simulink model "VA2_CV8_sim2017a"  (R2018a)
settings: Solver=ode45  StartTime=0.0  StopTime=3.5  RelTol=1e-3  EnableMultiTasking=on
values from neighbouring files (symbols this model uses):
  A = [ 0       1   0       0 ... (first row only)    [VA2_CV8_matlab_final.m]    (also in VA2_CV8_matlab_test.m)
  B = [0;    -0.0633;   0;   3.4960]    [VA2_CV8_matlab_final.m]    (also in VA2_CV8_matlab_test.m)
  C = eye(4)    [VA2_CV8_matlab_final.m]    (also in VA2_CV8_matlab_test.m)
  D = zeros(4,1)    [VA2_CV8_matlab_final.m]    (also in VA2_CV8_matlab_test.m)
  H = place(A', C', observer_poles)'    [VA2_CV8_matlab_final.m]
  Ki = -K(5)    [VA2_CV8_matlab_final.m]
  Kr = K(1:n)    [VA2_CV8_matlab_final.m]
  maxR = 7/weight    (= 1.29390018484)    [VA2_CV8_matlab_final.m]
libraries: sldrtlib x1
settings Model: Creator=pvel  LastModifiedBy=romanp
settings DataIOCC: LimitDataPoints=on  SaveFormat=Array
settings OptimizationCC: LifeSpan=inf
settings DebuggingCC: SFUnexpectedBacktrackingDiag=warning  SFNoUnconditionalDefaultTransitionDiag=warning  SFExecutionAtInitializationDiag=none
settings HardwareCC: ProdBitPerPointer=32  ProdBitPerSizeT=32  ProdBitPerPtrDiffT=32  ProdLargestAtomicFloat=None  ProdIntDivRoundTo=Undefined  ProdEndianess=Unspecified  ProdWordSize=32  ProdHWDeviceType=32-bit Generic
settings ModelReferenceCC: PropagateSignalLabelsOutOfModel=off
settings CodeAppCC: StateflowObjectComments=on
settings GRTTargetCC: TargetLangStandard=C89/C90 (ANSI)  GeneratePreprocessorConditionals=Disable all
settings ConfigComp: CovMetricSettings=dw  CovHtmlReporting=on  CovSaveCumulativeToWorkspaceVar=on  CovSaveSingleToWorkspaceVar=on  CovExternalEMLEnable=off

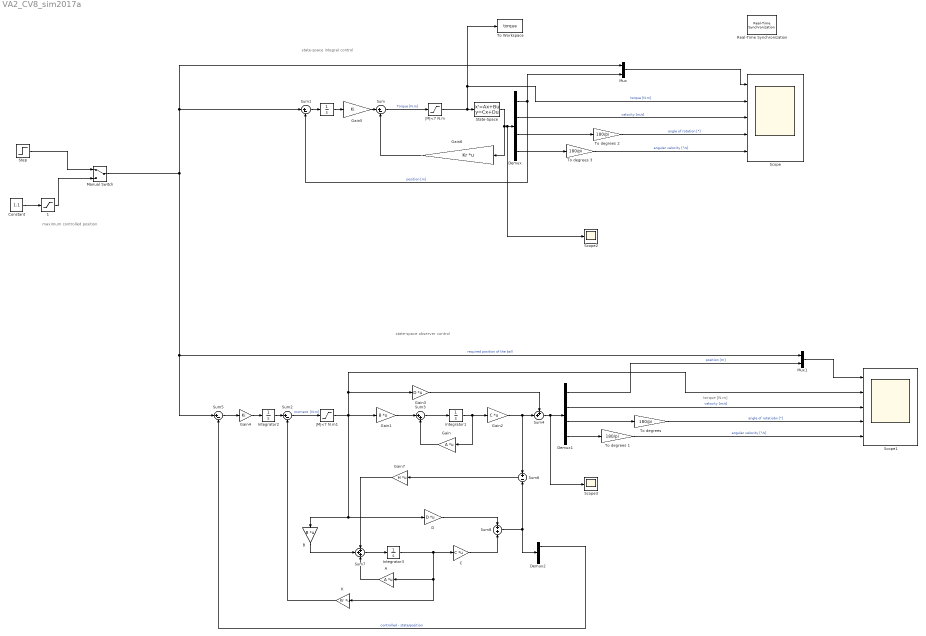
== system VA2_CV8_sim2017a ==
  note: torque [N.m]
  note: state-space integral control
  note: state-space observer control
  note: maximum controlled position
  " " : Integrator
  " 1" : Saturate  UpperLimit=maxR  LowerLimit=-maxR
  A : Gain  Gain=A  Multiplication=Matrix(K*u)
  B : Gain  Gain=B  Multiplication=Matrix(K*u)
  C : Gain  Gain=C  Multiplication=Matrix(K*u)
  Constant : Constant  Value=1.1
  "D " : Gain  Gain=D  Multiplication=Matrix(K*u)
  Demux : Demux
  Demux1 : Demux
  Demux2 : Demux
  Gain : Gain  Gain=A  Multiplication=Matrix(K*u)
  Gain1 : Gain  Gain=B  Multiplication=Matrix(K*u)
  Gain2 : Gain  Gain=C  Multiplication=Matrix(K*u)
  Gain3 : Gain  Gain=D  Multiplication=Matrix(K*u)
  Gain4 : Gain  Gain=Ki
  Gain5 : Gain  Gain=Ki
  Gain6 : Gain  Gain=Kr  Multiplication=Matrix(K*u) (u vector)
  Gain7 : Gain  Gain=H  Multiplication=Matrix(K*u)
  Integrator1 : Integrator
  Integrator2 : Integrator
  Integrator3 : Integrator
  K : Gain  Gain=Kr  Multiplication=Matrix(K*u)
  Manual Switch : ManualSwitch
  Mux : Mux  Inputs=2
  Mux1 : Mux  Inputs=2
  Real-Time Synchronization : sldrtlib/Real-Time Synchronization  SampleTime=0.1  MaxMissedTicks=10  ShowMissedTicks=off  YieldWhenWaiting=off
  Scope : Scope  NumInputPorts=5
  Scope1 : Scope  NumInputPorts=5
  Scope2 : Scope
  Scope3 : Scope
  State-Space : StateSpace  A=A  B=B  C=C  D=D  InitialCondition=0
  Step : Step  SampleTime=0
  Sum{,1..2,5} (4 alike) : Sum  Inputs=|+-
  Sum3 : Sum  Inputs=|++
  Sum4 : Sum  Inputs=++|
  Sum6 : Sum  Inputs=+-
  Sum7 : Sum  Inputs=+++
  Sum8 : Sum
  To Workspace : ToWorkspace  VariableName=torque  SaveFormat=Timeseries  SampleTime=-1
  To degrees : Gain  Gain=180/pi
  To degrees 1 : Gain  Gain=180/pi
  To degrees 2 : Gain  Gain=180/pi
  To degrees 3 : Gain  Gain=180/pi
  |M|<7 N.m : Saturate  UpperLimit=7  LowerLimit=-7
  |M|<7 N.m1 : Saturate  UpperLimit=7  LowerLimit=-7
  wires:
  Sum/1 -> |M|<7 N.m/1  "Torque [N.m]"
  Sum1/1 -> " "/1
  Demux/1 -> Mux/2, Sum1/2  "position [m]"
  Gain6/1 -> Sum/2
  " "/1 -> Gain5/1
  Gain5/1 -> Sum/1
  State-Space/1 -> Gain6/1, Scope2/1, Demux/1
  Demux/4 -> To degrees 3/1
  Step/1 -> Manual Switch/1
  Mux/1 -> Scope/1
  Demux/2 -> Scope/3  "velocity [m/s]"
  Demux/3 -> To degrees 2/1
  To degrees 2/1 -> Scope/4  "angle of rotation [°]"
  To degrees 3/1 -> Scope/5  "angular velocity [°/s]"
  |M|<7 N.m/1 -> To Workspace/1, Scope/2, State-Space/1  "torque [N.m]"
  Manual Switch/1 -> Mux/1, Sum1/1, Mux1/1, Sum5/1  "required position of the ball"
  Sum2/1 -> |M|<7 N.m1/1  "moment  [N.m]"
  Integrator1/1 -> Gain/1, Gain2/1
  Gain1/1 -> Sum3/1
  Sum3/1 -> Integrator1/1
  Gain/1 -> Sum3/2
  Gain2/1 -> Sum6/1, Sum4/2
  Gain3/1 -> Sum4/1
  Sum4/1 -> Scope3/1, Demux1/1
  Demux1/1 -> Mux1/2  "position [m]"
  Demux1/2 -> Scope1/3  "velocity [m/s]"
  Demux1/3 -> To degrees/1
  Demux1/4 -> To degrees 1/1
  Gain4/1 -> Integrator2/1
  Integrator2/1 -> Sum2/1
  Sum6/1 -> Gain7/1
  Gain7/1 -> Sum7/1
  B/1 -> Sum7/2
  Sum7/1 -> Integrator3/1
  Integrator3/1 -> K/1, A/1, C/1
  "D "/1 -> Sum8/1
  A/1 -> Sum7/3
  C/1 -> Sum8/2
  K/1 -> Sum2/2
  Sum8/1 -> Demux2/1, Sum6/2
  Demux2/1 -> Sum5/2  "controlled - state/position"
  Sum5/1 -> Gain4/1
  Mux1/1 -> Scope1/1
  To degrees 1/1 -> Scope1/5  "angular velocity [°/s]"
  To degrees/1 -> Scope1/4  "angle of rotatiobn [°]"
  |M|<7 N.m1/1 -> Gain1/1, Scope1/2, Gain3/1, B/1, "D "/1
  Constant/1 -> " 1"/1
  " 1"/1 -> Manual Switch/2
